simulink library "MuteControlBtc"  (R2022b)
settings: Solver=VariableStepAuto  StartTime=0.0  StopTime=10.0  RelTol=1e-3
libraries: FeaturePath x1, HandyTextFile x1, RTC x1, TuneVar x1
settings Model: Creator=kl13806  LastModifiedBy=kl13806
settings SolverCC: AlgebraicLoopSolver=TrustRegion
settings DebuggingCC: UnconnectedInputMsg=warning  UnconnectedOutputMsg=warning  UnconnectedLineMsg=warning  SFMachineParentedDataDiag=warning
settings ModelReferenceCC: EnableRefExpFcnMdlSchedulingChecks=on
settings RTWCC: DLArmComputeVersion=19.05

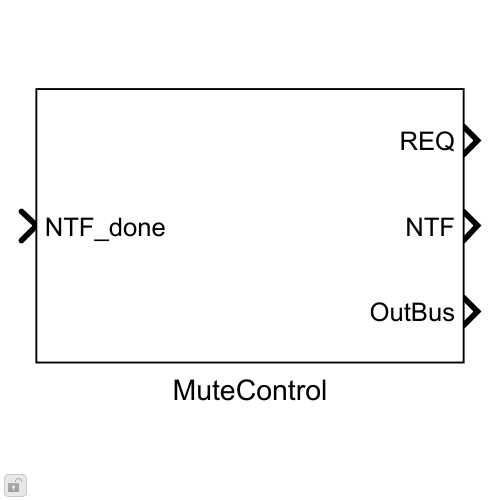
[thumbnail: Simulink's stored preview of the top-level diagram]
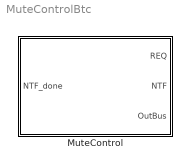
== system MuteControlBtc ==
  MuteControl : Subsystem  mask(Blocklib MuteControl){Config=[], FeatureName=MuteControl}
      mask prompts: Config "MuteControlConfig"; FeatureName "Mask feature name:"
      mask help: This component is to be used in conjunction with 1 or more instances of the MuteRamper block. There is no mask for this component. It provides the control layer for Mute processing via an RTC and tune variable, muteControlRampTime.
      mask init:
      | blkh=gcbh;
      | Config=BTConfig.Assert(blkh,Config);
      | BTConfig.InitSetFeatureIfPresent(blkh,'FeatureName');
      | Config.Validate();
      | 
      | % Set boundary conditions
      | rampRateBounds = [5,50000];
      | rampTimeBounds = [1,3000];
      mask Help: If this control block is being used in a "multi-instance" manner, i.e. it is contorlling two or more MuteRamper blocks, there is an additional step that must be done. The developer must add a function-triggered subsytem containing an AND logic gate, which will combine the notification completion signals of the multiple ramper instances. The output of this subsytem must then feed the NTF_done input of the MuteControl block.
      mask Callback Config: BTConfig.CallbackHideIfPresent(gcbh,{'FeatureName'});
      mask TypeOptions FeatureName: FeaturePath/FeatureName

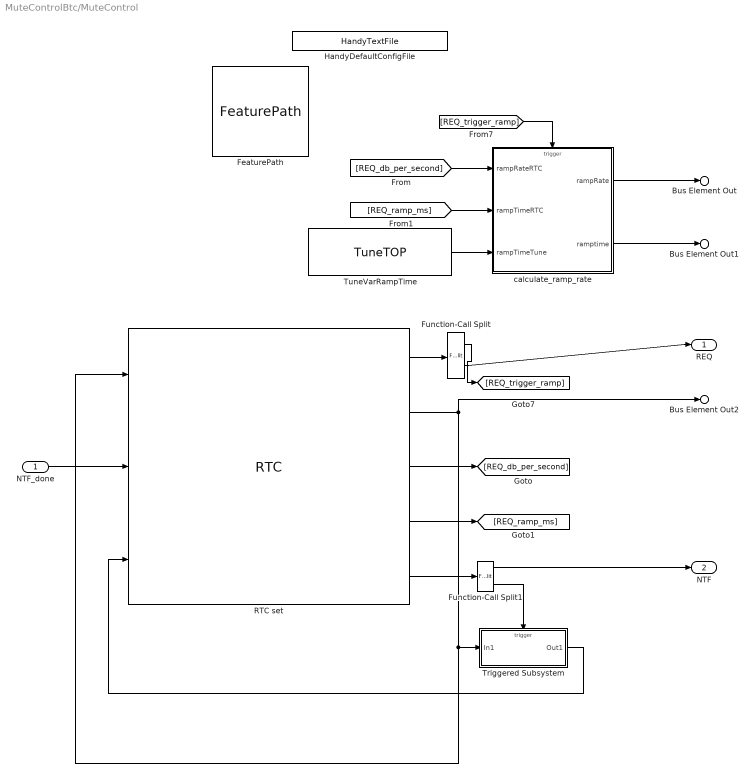
== system MuteControlBtc/MuteControl ==
  NTF_done : Inport
  FeaturePath : FeaturePath/FeaturePath  FeatureName=MuteControl  IsGroup=off  GroupNumber=-1  IsModule=off  TriggerInit=[180 39 295 146]
      settings: SourceProductName=Bose Talaria
  Function-Call Split : FunctionCallSplit  IconShape=distinctive  NumOutputPorts=2
  Function-Call Split1 : FunctionCallSplit  IconShape=distinctive  NumOutputPorts=2  OutputPortLayout=default
  HandyDefaultConfigFile : HandyTextFile/HandyTextFile  TemplateSource=Config  FileSuffix=Init  OpenDialogOnLoad=off  UseThisBlockName=off  AddGrandParentNamePrefix=off  TheDefaultText=|  ShowInLibBrowser=on
      | % $(FILENAME) Setup model parameters for each "Init" callback (e.g. update diagram)
      | sample_rate_in_hertz = 44100;
      | frame_size = 32;
      | sysin_channel_count = 2;
      settings: SourceProductName=Bose Talaria
  RTC set : RTC/RTC  Description="Command a mute by specifying whether mute is active (non zero mute_switch) or inactive (mute_switch is \"0\"). If db_per_second is non-zero, it commands the timing of the mute, otherwise the ramp_milliseconds is used."  REQ_Priority=RTC_Mask.NormalPriority  RequestAtInit=off  EnableRequest=on  REQElemName1=mute_switch  REQElemType1=uint32  REQElemWidth1=1  REQElemInitial1=[]  REQElemName2=ramp_db_per_second  REQElemType2=uint32  REQElemWidth2=1  REQElemInitial2=[]  REQElemName3=ramp_milliseconds  REQElemType3=uint32  REQElemWidth3=1  REQElemInitial3=[]  REQElemType4=uint32  REQElemWidth4=1  REQElemInitial4=[]  REQElemType5=uint32  REQElemWidth5=1  REQElemInitial5=[]  REQElemType6=uint32  REQElemWidth6=1  REQElemInitial6=[]  REQElemType7=uint32  REQElemWidth7=1  REQElemInitial7=[]  REQElemType8=uint32  REQElemWidth8=1  REQElemInitial8=[]  REQElemType9=uint32  REQElemWidth9=1  REQElemInitial9=[]  REQElemType10=uint32  REQElemWidth10=1  REQElemInitial10=[]  EnableResponse=on  EnableRSP_StatusIn=off  RSPElemName1=mute_switch  RSPElemType1=uint32  RSPElemWidth1=1  RSPElemType2=uint32  RSPElemWidth2=1  RSPElemType3=uint32  RSPElemWidth3=1  RSPElemType4=uint32  RSPElemWidth4=1  RSPElemType5=uint32  RSPElemWidth5=1  RSPElemType6=uint32  RSPElemWidth6=1  RSPElemType7=uint32  RSPElemWidth7=1  RSPElemType8=uint32  RSPElemWidth8=1  RSPElemType9=uint32  RSPElemWidth9=1  RSPElemType10=uint32  RSPElemWidth10=1  EnableNotification=on  EnableNTF_PrepTrig=off  NTFElemName1=mute_switch  NTFElemType1=uint32  NTFElemWidth1=1  NTFElemType2=uint32  NTFElemWidth2=1  NTFElemType3=uint32  NTFElemWidth3=1  NTFElemType4=uint32  NTFElemWidth4=1  NTFElemType5=uint32  NTFElemWidth5=1  NTFElemType6=uint32  NTFElemWidth6=1  NTFElemType7=uint32  NTFElemWidth7=1  NTFElemType8=uint32  NTFElemWidth8=1  NTFElemType9=uint32  NTFElemWidth9=1  NTFElemType10=uint32  NTFElemWidth10=1  MaskMessageName=Set
      settings: SourceProductName=Bose Talaria
  Triggered Subsystem : Subsystem  TreatAsAtomicUnit=on
  TuneVarRampTime : TuneVar/TuneTOP  Description=|  TriggerInit=[295 232 465 288]  TopName=RampTime  TuneName=RampTime  DataType=single  TunabilityNumber=1  MinValue=1  MaxValue=100000  BankNumber=0  PreOverlay=false  PostOverlay=false  UseSameName=on  MaskValue=Config.DefaultRampTimeMsec
      | Specifies the default value of ramp time for the Mute or Unmute operation.
      | Used only when the RTC message does not contain either ramp rate or ramp time.
      settings: SourceProductName=Bose Talaria
  calculate_ramp_rate : MATLAB Function  TreatAsAtomicUnit=on
  REQ : Outport
  NTF : Outport  Port=2
  Bus Element Out : Outport  Port=3  PortName=OutBus  Element=rampRate
  Bus Element Out1 : Outport  Port=3  PortName=OutBus  Element=rampTime
  Bus Element Out2 : Outport  Port=3  PortName=OutBus  Element=REQ_mute_switch
  wires:
  Function-Call Split/2 -> REQ/1
  calculate_ramp_rate/2(ramptime) -> Bus Element Out1/1
  NTF_done/1 -> RTC set/2
  RTC set/4 -> [REQ_ramp_ms]
  RTC set/3 -> [REQ_db_per_second]
  Triggered Subsystem/1(Out1) -> RTC set/3
  [REQ_ramp_ms] -> calculate_ramp_rate/2(rampTimeRTC)
  calculate_ramp_rate/1(rampRate) -> Bus Element Out/1
  TuneVarRampTime/1 -> calculate_ramp_rate/3(rampTimeTune)
  RTC set/1 -> Function-Call Split/1
  Function-Call Split/1 -> [REQ_trigger_ramp]
  [REQ_trigger_ramp] -> calculate_ramp_rate/Trigger
  RTC set/5 -> Function-Call Split1/1
  Function-Call Split1/2 -> Triggered Subsystem/Trigger
  Function-Call Split1/1 -> NTF/1
  [REQ_db_per_second] -> calculate_ramp_rate/1(rampRateRTC)
  RTC set/2 -> RTC set/1, Triggered Subsystem/1(In1), Bus Element Out2/1

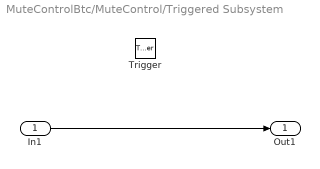
== system MuteControlBtc/MuteControl/Triggered Subsystem ==
  In1 : Inport
  Trigger : TriggerPort  TriggerType=function-call  VariantControl=Variant
  Out1 : Outport
  wires:
  In1/1 -> Out1/1

== matlab function MuteControlBtc/MuteControl/calculate_ramp_rate ==
  data: rampRateRTC input; rampRate output; rampTimeRTC input; ramptime output; rampTimeTune input; rampRateBounds parameter; rampTimeBounds parameter
  events: trigger input FUNCTION_CALL_EVENT
function [rampRate,ramptime] = Calculate_ramp_parameters(rampRateRTC, rampTimeRTC, rampTimeTune,... % Inputs
    rampRateBounds, rampTimeBounds) % parameters

% Ramp time and rate are provided to the block through RTC messages. However 
% in case neither of them are provided, the block will use the default ramp 
% time given in the tune variable.

    ramptime = single(rampTimeTune);
    rampRate = single(0);
    
    if (rampRateRTC)
        rampRate = single(rampRateRTC);
        rampRate = max(rampRateBounds(1), rampRate);
        rampRate = min(rampRateBounds(2), rampRate);
    end
    if (rampTimeRTC)
        ramptime = single(rampTimeRTC);
    end
    ramptime = max(rampTimeBounds(1), ramptime);
    ramptime = min(rampTimeBounds(2), ramptime);
end
